simulink model "solarpanel_motor_position_tracking"  (R2021b)
settings: Solver=VariableStepAuto  StartTime=0.0  StopTime=20  RelTol=1e-3
libraries: slpidlib x1
settings Model: Creator=mprad  LastModifiedBy=mprad

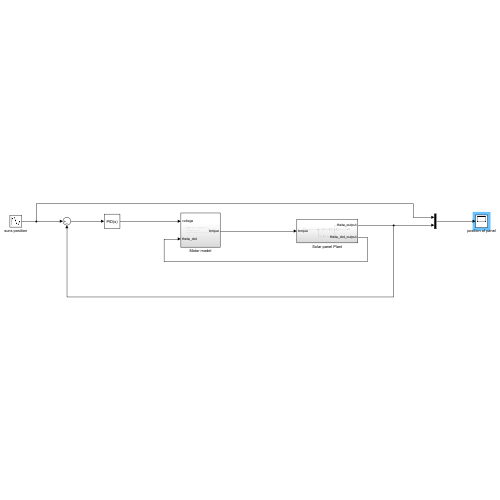
[thumbnail: Simulink's stored preview of the top-level diagram]
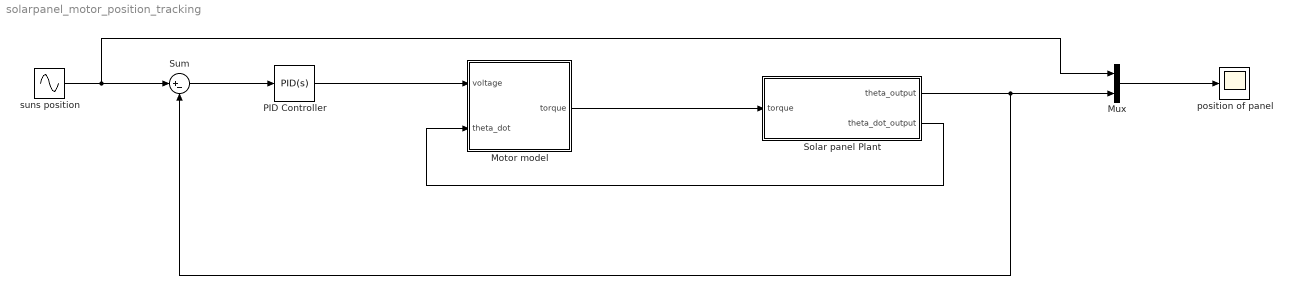
== system solarpanel_motor_position_tracking ==
  Motor model : Subsystem
  Mux : Mux  Inputs=2
  PID Controller : slpidlib/PID Controller  Controller=PID  Form=Parallel  TimeDomain=Continuous-time  UseExternalTs=off  SampleTime=-1  IntegratorMethod=Forward Euler  FilterMethod=Forward Euler  ControllerParametersSource=internal  P=8.0394415799935  I=3.41112454090938  D=2.02693786658582  UseFilter=on  N=562.102722544759  TunerSelectOption=Transfer Function Based (PID Tuner App)  InitialConditionSource=internal  InitialConditionForIntegrator=0  InitialConditionForFilter=0  DifferentiatorICPrevScaledInput=0  ExternalReset=none  TrackingMode=off  Kt=1  LimitOutput=off  SatLimitsSource=internal  UpperSaturationLimit=inf  LowerSaturationLimit=-inf  LinearizeAsGain=on  AntiWindupMode=none  Kb=1  POutMin=[]  POutMax=[]  IOutMin=[]  IOutMax=[]  DOutMin=[]  DOutMax=[]  NOutMin=[]  NOutMax=[]  SumOutMin=[]  SumOutMax=[]  SaturationOutMin=[]  SaturationOutMax=[]  PParamMin=[]  PParamMax=[]  IParamMin=[]  IParamMax=[]  DParamMin=[]  DParamMax=[]  NParamMin=[]  NParamMax=[]  KbParamMin=[]  KbParamMax=[]  KtParamMin=[]  KtParamMax=[]  KbOutMin=[]  KbOutMax=[]  KtOutMin=[]  KtOutMax=[]  IntegratorOutMin=[]  IntegratorOutMax=[]  FilterOutMin=[]  FilterOutMax=[]  SumI1OutMin=[]  SumI1OutMax=[]  SumI2OutMin=[]  SumI2OutMax=[]  SumI3OutMin=[]  SumI3OutMax=[]  SumI4OutMin=[]  SumI4OutMax=[]  SumDOutMin=[]  SumDOutMax=[]  DifferentiatorOutMin=[]  DifferentiatorOutMax=[]  FilterDiffOutCoefMin=[]  FilterDiffOutCoefMax=[]  ReciprocalOutMin=[]  ReciprocalOutMax=[]  SumDenOutMin=[]  SumDenOutMax=[]  SumNumOutMin=[]  SumNumOutMax=[]  DivideOutMin=[]  DivideOutMax=[]  UdiffTsProdOutMin=[]  UdiffTsProdOutMax=[]  NTsProdOutMin=[]  NTsProdOutMax=[]  UintegralTsProdOutMin=[]  UintegralTsProdOutMax=[]  UngainTsProdOutMin=[]  UngainTsProdOutMax=[]  IntegratorContinuousStateAttributes=''  IntegratorStateMustResolveToSignalObject=off  IntegratorRTWStateStorageClass=Auto  FilterContinuousStateAttributes=''  FilterStateMustResolveToSignalObject=off  FilterRTWStateStorageClass=Auto  ParallelPVariant=InternalParameters  IdealPVariant=Disabled  IVariant=InternalParameters  DVariant=InternalParameters  IntegratorVariant=Continuous  SatVariant=Disabled  AWVariant=Passthrough  PCopyVariant=Disabled  TRVariant=Disabled  FdbkBlocksVariant=Forward  IdealPFdbkVariant=Disabled  SatFdbkVariant=Disabled  DerivativeFilterVariant=ContFilter  NVariant=InternalParameters  NCopyVariant=Disabled  FilterICVariant=InternalICsFilter  IntegratorICVariant=InternalICs  ExternalResetVariant=Disabled  TRSumVariant=Passthrough  SumFdbkVariant=Disabled  SumVariant=Sum_PID  TsampFilterVariant=InternalTs  TsampNgainVariant=Passthrough  TsampIntegralVariant=Passthrough  ExternalSaturationOutDataTypeStr=Inherit: Same as second input
  Solar panel Plant : Subsystem
  Sum : Sum  Inputs=|+-
  position of panel : Scope
  suns position : Sin  Amplitude=0.5  Frequency=0.75  SampleTime=0
  wires:
  Solar panel Plant/2(theta_dot_output) -> Motor model/2(theta_dot)
  Motor model/1(torque) -> Solar panel Plant/1(torque)
  Solar panel Plant/1(theta_output) -> Mux/2, Sum/2
  suns position/1 -> Mux/1, Sum/1
  Sum/1 -> PID Controller/1
  PID Controller/1 -> Motor model/1(voltage)
  Mux/1 -> position of panel/1

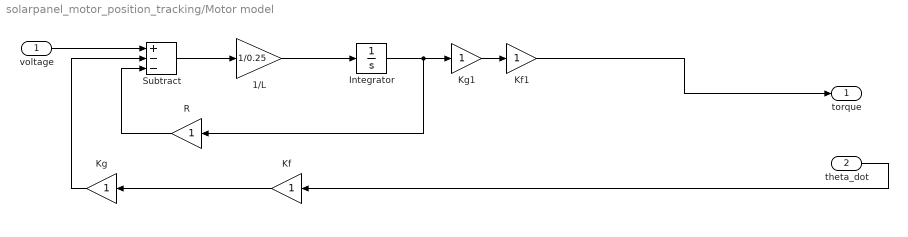
== system solarpanel_motor_position_tracking/Motor model ==
  voltage : Inport
  theta_dot : Inport  Port=2
  1/L : Gain  Gain=1/0.25
  Integrator : Integrator
  Kf : Gain
  Kf1 : Gain
  Kg : Gain
  Kg1 : Gain
  R : Gain
  Subtract : Sum  Inputs=+--
  torque : Outport
  wires:
  Integrator/1 -> Kg1/1, R/1
  Kf/1 -> Kg/1
  Kg1/1 -> Kf1/1
  1/L/1 -> Integrator/1
  Subtract/1 -> 1/L/1
  Kg/1 -> Subtract/2
  voltage/1 -> Subtract/1
  R/1 -> Subtract/3
  theta_dot/1 -> Kf/1
  Kf1/1 -> torque/1

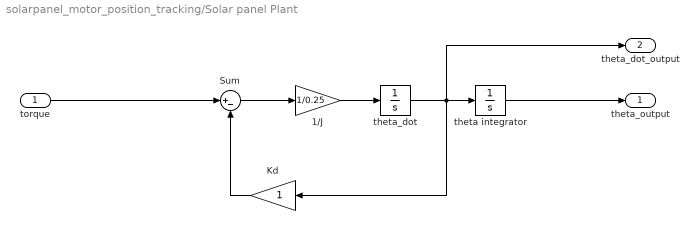
== system solarpanel_motor_position_tracking/Solar panel Plant ==
  torque : Inport
  1/J : Gain  Gain=1/0.25
  Kd : Gain
  Sum : Sum  Inputs=|+-
  theta integrator : Integrator
  theta_dot : Integrator
  theta_output : Outport
  theta_dot_output : Outport  Port=2
  wires:
  torque/1 -> Sum/1
  Sum/1 -> 1/J/1
  theta_dot/1 -> theta_dot_output/1, Kd/1, theta integrator/1
  1/J/1 -> theta_dot/1
  Kd/1 -> Sum/2
  theta integrator/1 -> theta_output/1
